simulink model "lab8"  (R2014b)
settings: Solver=ode45  StartTime=0.0  StopTime=150  RelTol=1e-3
libraries: simulink x4, fuzblock x4
settings Model: Creator=StudentPA  LastModifiedBy=StudentPA

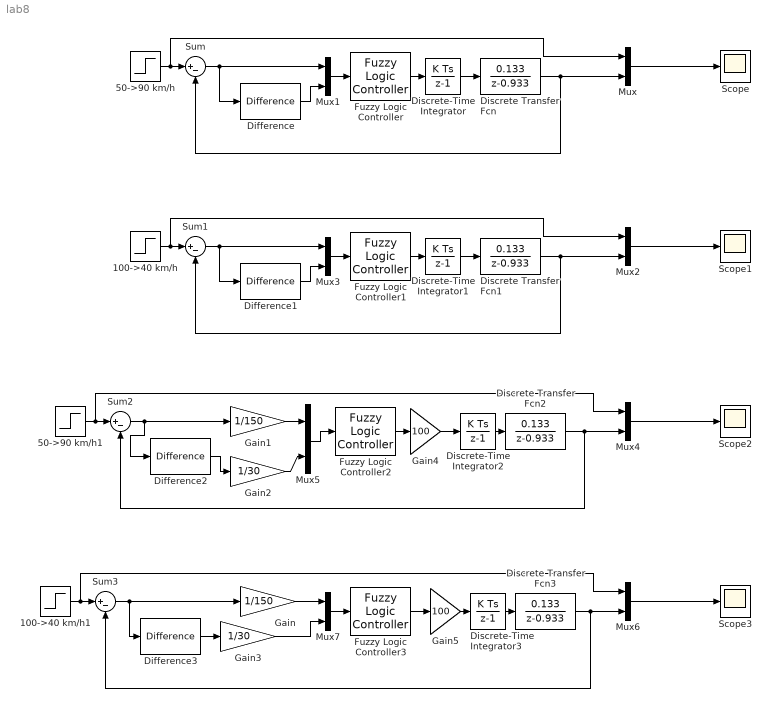
== system lab8 ==
  100->40 km/h : Step  Before=100  After=40  SampleTime=1
  100->40 km/h1 : Step  Before=100  After=40  SampleTime=1
  50->90 km/h : Step  Before=50  After=90  SampleTime=1
  50->90 km/h1 : Step  Before=50  After=90  SampleTime=1
  Difference{,1..3} (4 alike) : simulink/Discrete/Difference  ICPrevInput=0.0  InputProcessing=Inherited  OutMin=[]  OutMax=[]  OutDataType=fixdt(1, 16)  OutScaling=2^-10  DoSatur=off
  Discrete Transfer Fcn{,1..3} (4 alike) : DiscreteTransferFcn  Numerator=[0.133]  Denominator=[1 -0.933]  SampleTime=1
  Discrete-Time Integrator{,1..3} (4 alike) : DiscreteIntegrator  InitialConditionSetting=State (most efficient)
  Fuzzy Logic Controller : fuzblock/Fuzzy Logic  Controller  fis=nieznormal
  Fuzzy Logic Controller1 : fuzblock/Fuzzy Logic  Controller  fis=nieznormal
  Fuzzy Logic Controller2 : fuzblock/Fuzzy Logic  Controller  fis=znormal
  Fuzzy Logic Controller3 : fuzblock/Fuzzy Logic  Controller  fis=znormal
  Gain : Gain  Gain=1/150
  Gain1 : Gain  Gain=1/150
  Gain2 : Gain  Gain=1/30
  Gain3 : Gain  Gain=1/30
  Gain4 : Gain  Gain=100
  Gain5 : Gain  Gain=100
  Mux{,1..7} (8 alike) : Mux  Inputs=2
  Scope{,1..3} (4 alike) : Scope
      Scope settings: ShowLegends=on
      Scope1 settings: ShowLegends=on
      Scope2 settings: ShowLegends=on  SaveName=ScopeData2
      Scope3 settings: ShowLegends=on  SaveName=ScopeData3
  Sum{,1..3} (4 alike) : Sum  Inputs=|+-
  wires:
  Mux1/1 -> Fuzzy Logic Controller/1
  Sum/1 -> Difference/1, Mux1/1
  50->90 km/h/1 -> Mux/1, Sum/1
  Discrete Transfer Fcn/1 -> Mux/2, Sum/2
  Difference/1 -> Mux1/2
  Mux/1 -> Scope/1
  Mux3/1 -> Fuzzy Logic Controller1/1
  Sum1/1 -> Mux3/1, Difference1/1
  100->40 km/h/1 -> Mux2/1, Sum1/1
  Discrete Transfer Fcn1/1 -> Sum1/2, Mux2/2
  Difference1/1 -> Mux3/2
  Mux2/1 -> Scope1/1
  Fuzzy Logic Controller/1 -> Discrete-Time Integrator/1
  Discrete-Time Integrator/1 -> Discrete Transfer Fcn/1
  Fuzzy Logic Controller1/1 -> Discrete-Time Integrator1/1
  Discrete-Time Integrator1/1 -> Discrete Transfer Fcn1/1
  Mux5/1 -> Fuzzy Logic Controller2/1
  Sum2/1 -> Gain1/1, Difference2/1
  50->90 km/h1/1 -> Sum2/1, Mux4/1
  Discrete Transfer Fcn2/1 -> Sum2/2, Mux4/2
  Difference2/1 -> Gain2/1
  Mux4/1 -> Scope2/1
  Mux7/1 -> Fuzzy Logic Controller3/1
  Sum3/1 -> Difference3/1, Gain/1
  100->40 km/h1/1 -> Sum3/1, Mux6/1
  Discrete Transfer Fcn3/1 -> Sum3/2, Mux6/2
  Difference3/1 -> Gain3/1
  Mux6/1 -> Scope3/1
  Discrete-Time Integrator2/1 -> Discrete Transfer Fcn2/1
  Discrete-Time Integrator3/1 -> Discrete Transfer Fcn3/1
  Gain/1 -> Mux7/1
  Gain1/1 -> Mux5/1
  Gain2/1 -> Mux5/2
  Gain3/1 -> Mux7/2
  Fuzzy Logic Controller2/1 -> Gain4/1
  Gain4/1 -> Discrete-Time Integrator2/1
  Fuzzy Logic Controller3/1 -> Gain5/1
  Gain5/1 -> Discrete-Time Integrator3/1
